simulink model "exam"  (R2019b)
settings: Solver=ode1  StartTime=0.0  StopTime=10  FixedStep=0.001  RelTol=1e-3
values from neighbouring files (symbols this model uses):
  A = [18  0  0; -1  10  3; 2  0  5]    [exam.mat]
  A2 = sys.a-sys.b*k    [exam.m]    (also in exam.mat = [-18  -3.34375  -0.41015625; 32  0  0; 0  16  0])
  Ac = [0  1  0; 0  0  1; -10  -5  8]    [exam.mat]
  B = [0 7 0]    [exam.mat]
  Bc = [0 0 1]    [exam.mat]
  C = [2 3 0]    [exam.mat]
  k = acker(sys.A,sys.B, [-3 -4 -5])    [exam.m]    (also in exam.mat = [30 58.3125 29.921875])
  k2 = -1.62162162162    [exam.mat]
  kc = 10    [exam.mat]
  kd = 0.5    [exam.mat]
  ki = 3.91061452514    [exam.mat]
  L = [1820.94972067 1276.72253259 307.48603352]    [exam.mat]
  sys = ss(G)    [exam.m]
undefined symbols (not defined in the file or in its folder): sysG
libraries: cstblocks x7, simulink x2
settings Model: Creator=Dell  LastModifiedBy=Dell

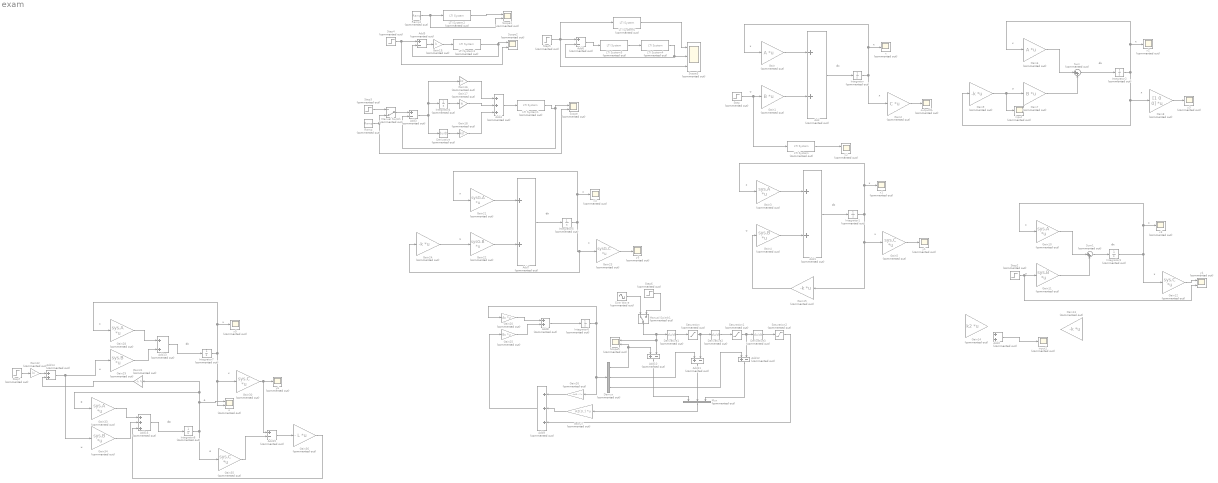
== system exam ==
  note: dx
  note: x
  note: x
  note: dx
  note: x
  note: x
  note: x
  note: x
  note: u
  note: u
  note: u
  note: x
  note: x
  note: dx
  note: x
  note: x
  note: x
  note: x
  note: x
  note: u
  note: x
  note: x
  note: dx
  note: u
  note: dx
  note: x
  note: x
  note: dx
  note: u
  note: x
  note: o
  note: o
  note: o
  note: do
  note: u
  Add{,1..2,7..8,13..14} (7 alike) : Sum  Commented=on
  Add{3,5..6,10..12,15} (7 alike) : Sum  Commented=on  Inputs=+-
  Add16 : Sum  Commented=on  Inputs=+++
  Add4 : Sum  Commented=on  Inputs=+++
  Add9 : Sum  Commented=on  Inputs=+++
  Demux : Demux  Commented=on  Outputs=3
  Derivative{,1..3} (4 alike) : Derivative  Commented=on
  Gain : Gain  Commented=on  Gain=A  Multiplication=Matrix(K*u)
  Gain1 : Gain  Commented=on  Gain=B  Multiplication=Matrix(K*u)
  Gain{3,10,28,33} (4 alike) : Gain  Commented=on  Gain=sys.A  Multiplication=Matrix(K*u)
  Gain{4,11,29,34} (4 alike) : Gain  Commented=on  Gain=sys.B  Multiplication=Matrix(K*u)
  Gain{5,12,30,35} (4 alike) : Gain  Commented=on  Gain=sys.C  Multiplication=Matrix(K*u)
  Gain{9,13,15,24,31} (5 alike) : Gain  Commented=on  Gain=-k  Multiplication=Matrix(K*u)
  Gain14 : Gain  Commented=on  Gain=k2  Multiplication=Matrix(K*u)
  Gain16 : Gain  Commented=on  Gain=kc
  Gain17 : Gain  Commented=on  Gain=ki
  Gain18 : Gain  Commented=on  Gain=kd
  Gain19 : Gain  Commented=on  Gain=k
  Gain2 : Gain  Commented=on  Gain=C  Multiplication=Matrix(K*u)
  Gain20 : Gain  Commented=on  Gain=Ac  Multiplication=Matrix(K*u)
  Gain21 : Gain  Commented=on  Gain=sysG.A  Multiplication=Matrix(K*u)
  Gain22 : Gain  Commented=on  Gain=sysG.B  Multiplication=Matrix(K*u)
  Gain23 : Gain  Commented=on  Gain=sysG.C  Multiplication=Matrix(K*u)
  Gain25 : Gain  Commented=on  Gain=Bc  Multiplication=Matrix(K*u)
  Gain26 : Gain  Commented=on  Gain=-Ac(3,:)  Multiplication=Matrix(K*u)
  Gain27 : Gain  Commented=on  Gain=A2(3,:)  Multiplication=Matrix(K*u)
  Gain32 : Gain  Commented=on  Gain=ki
  Gain36 : Gain  Commented=on  Gain=- L  Multiplication=Matrix(K*u)
  Gain6 : Gain  Commented=on  Gain=A  Multiplication=Matrix(K*u)
  Gain7 : Gain  Commented=on  Gain=B  Multiplication=Matrix(K*u)
  Gain8 : Gain  Commented=on  Gain=[1 0 0]  Multiplication=Matrix(K*u)
  Integrator : Integrator  Commented=on
  Integrator{1..2,5,7..8} (5 alike) : Integrator  Commented=on  InitialCondition=[1 0 0]
  Integrator3 : Integrator  Commented=on  InitialCondition=[1 5 16]
  Integrator4 : Integrator  Commented=on
  Integrator6 : Integrator  Commented=on
  LTI System{,3..4,6} (4 alike) : cstblocks/LTI System  Commented=on  sys=G  IC=[]
  LTI System1 : cstblocks/LTI System  Commented=on  sys=G5  IC=[]
  LTI System2 : cstblocks/LTI System  Commented=on  sys=G5  IC=[]
  LTI System5 : cstblocks/LTI System  Commented=on  sys=C  IC=[]
  Manual Switch : ManualSwitch  Commented=on  CurrentSetting=0
  Manual Switch1 : ManualSwitch  Commented=on
  Mux : Mux  Commented=on  Inputs=3
  Ramp : simulink/Sources/Ramp  Commented=on  slope=7  start=0  InitialOutput=0
  Ramp1 : simulink/Sources/Ramp  Commented=on  slope=7  start=0  InitialOutput=0
  Saturation : Saturate  Commented=on  UpperLimit=3  LowerLimit=-3
  Saturation1 : Saturate  Commented=on  UpperLimit=3  LowerLimit=-3
  Saturation2 : Saturate  Commented=on  UpperLimit=3  LowerLimit=-3
  Scope{,1..2,5} (4 alike) : Scope  Commented=on  NumInputPorts=2
  Scope3 : Scope  Commented=on  NumInputPorts=3
  Sine Wave : Sin  Commented=on  Amplitude=3  SampleTime=0
  Step{,3..5} (4 alike) : Step  Commented=on  Time=0  SampleTime=0
  Step2 : Step  Commented=on  Time=0  After=2  SampleTime=0
  Step6 : Step  Commented=on  SampleTime=0
  Step7 : Step  Commented=on  Time=0  After=4  SampleTime=0
  Sum : Sum  Commented=on  Inputs=|++
  Sum1 : Sum  Commented=on  Inputs=|++
  input : Scope  Commented=on
  input1 : Scope  Commented=on
  o : Scope  Commented=on  NumInputPorts=2
  outputOL : Scope  Commented=on
  x{,1..5} (6 alike) : Scope  Commented=on
  y{1,3,5..6} (4 alike) : Scope  Commented=on
  y2 : Scope  Commented=on  NumInputPorts=2
  y4 : Scope  Commented=on  NumInputPorts=2
  wires:
  Add6/1 -> LTI System5/1
  Step5/1 -> LTI System6/1, Scope3/3, Add6/1
  Step4/1 -> Scope2/2, Add5/1
  LTI System3/1 -> Add5/2, Scope2/1
  Gain18/1 -> Add4/3
  Derivative/1 -> Gain18/1
  Step3/1 -> Manual Switch/1
  Gain17/1 -> Add4/2
  LTI System2/1 -> Scope1/1
  Add4/1 -> LTI System1/1
  Gain23/1 -> y5/1
  Add7/1 -> Integrator5/1
  Integrator5/1 -> x4/1, Gain21/1, Gain24/1, Gain23/1
  Gain22/1 -> Add7/2
  Add1/1 -> Integrator1/1
  Sum1/1 -> Integrator3/1
  Integrator1/1 -> x1/1, Gain3/1, Gain15/1, Gain5/1
  Gain24/1 -> Gain22/1
  Gain9/1 -> input/1, Gain7/1
  Gain8/1 -> y3/1
  Gain10/1 -> Sum1/1
  Gain12/1 -> y4/1
  Gain2/1 -> outputOL/1
  Integrator2/1 -> x2/1, Gain6/1, Gain9/1, Gain8/1
  Add2/1 -> input1/1
  Gain7/1 -> Sum/2
  Gain4/1 -> Add1/2
  Integrator/1 -> x/1, Gain/1, Gain2/1
  Gain1/1 -> Add/2
  Integrator3/1 -> x3/1, Gain10/1, Gain12/1
  Gain3/1 -> Add1/1
  Sum/1 -> Integrator2/1
  LTI System/1 -> y2/1
  Step/1 -> LTI System/1, Gain1/1
  Add3/1 -> Derivative/1, Integrator4/1, Gain16/1
  Gain5/1 -> y1/1
  Gain16/1 -> Add4/1
  LTI System6/1 -> Scope3/1
  Ramp/1 -> Manual Switch/2, Scope/2
  LTI System4/1 -> Scope3/2, Add6/2
  Gain19/1 -> LTI System3/1
  Manual Switch/1 -> Add3/1
  LTI System1/1 -> Add3/2, Scope/1
  Add5/1 -> Gain19/1
  Gain11/1 -> Sum1/2
  Ramp1/1 -> Scope1/2, LTI System2/1
  Add/1 -> Integrator/1
  Gain21/1 -> Add7/1
  LTI System5/1 -> LTI System4/1
  Integrator4/1 -> Gain17/1
  Gain6/1 -> Sum/1
  Gain/1 -> Add/1
  Gain20/1 -> Add8/1
  Add8/1 -> Integrator6/1
  Gain25/1 -> Add8/2
  Integrator6/1 -> Gain20/1, Demux/1, Gain26/1
  Gain26/1 -> Add9/1
  Add9/1 -> Gain25/1
  Sine Wave/1 -> Manual Switch1/1
  Step6/1 -> Manual Switch1/2
  Derivative1/1 -> Saturation/1
  Derivative2/1 -> Saturation1/1
  Saturation/1 -> Add11/2, Derivative2/1
  Derivative3/1 -> Saturation2/1
  Saturation1/1 -> Add12/2, Derivative3/1
  Demux/1 -> Scope5/2, Add10/1
  Demux/2 -> Add11/1
  Demux/3 -> Add12/1
  Add12/1 -> Mux/3
  Add11/1 -> Mux/2
  Add10/1 -> Mux/1
  Mux/1 -> Gain27/1
  Gain27/1 -> Add9/2
  Saturation2/1 -> Add9/3
  Manual Switch1/1 -> Scope5/1, Add10/2, Derivative1/1
  Gain28/1 -> Add13/1
  Gain29/1 -> Add13/2
  Gain30/1 -> Add15/1, y6/1
  Integrator7/1 -> x5/1, Gain28/1, o/2, Gain30/1
  Add13/1 -> Integrator7/1
  Gain32/1 -> Add14/1
  Step7/1 -> Gain32/1
  Add14/1 -> Gain34/1, Gain29/1
  Add16/1 -> Integrator8/1
  Integrator8/1 -> o/1, Gain31/1, Gain33/1, Gain35/1
  Gain33/1 -> Add16/1
  Gain35/1 -> Add15/2
  Gain34/1 -> Add16/2
  Add15/1 -> Gain36/1
  Gain36/1 -> Add16/3
  Gain31/1 -> Add14/2
  Step2/1 -> y4/2, Gain11/1
  Gain15/1 -> Gain4/1
